simulink model "DDC_MPTC"  (R2023b)
settings: Solver=FixedStepDiscrete  StartTime=0.0  StopTime=0.5  RelTol=1e-3
libraries: spsGroundLib x1, spsPermanentMagnetSynchronousMachineLib x1, simulink x1, spsUniversalBridgeLib x1, spsDCVoltageSourceLib x1, slpidlib x1, spspowerguiLib x1
settings Model: Creator=蓝轩  LastModifiedBy=rainy
settings SolverCC: AlgebraicLoopSolver=TrustRegion
settings DataIOCC: ReturnWorkspaceOutputs=off
settings DebuggingCC: UnconnectedInputMsg=warning  UnconnectedOutputMsg=warning  UnconnectedLineMsg=warning  ArithmeticOperatorsInVariantConditions=warning
settings ModelReferenceCC: EnableRefExpFcnMdlSchedulingChecks=on
settings SFSimCC: CustomCodeUndefinedFunction=UseInterfaceOnly

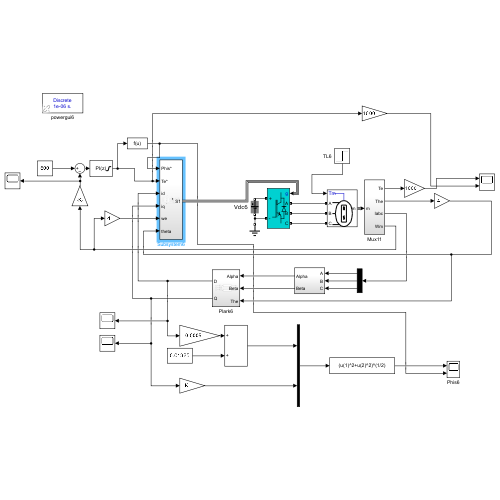
[thumbnail: Simulink's stored preview of the top-level diagram]
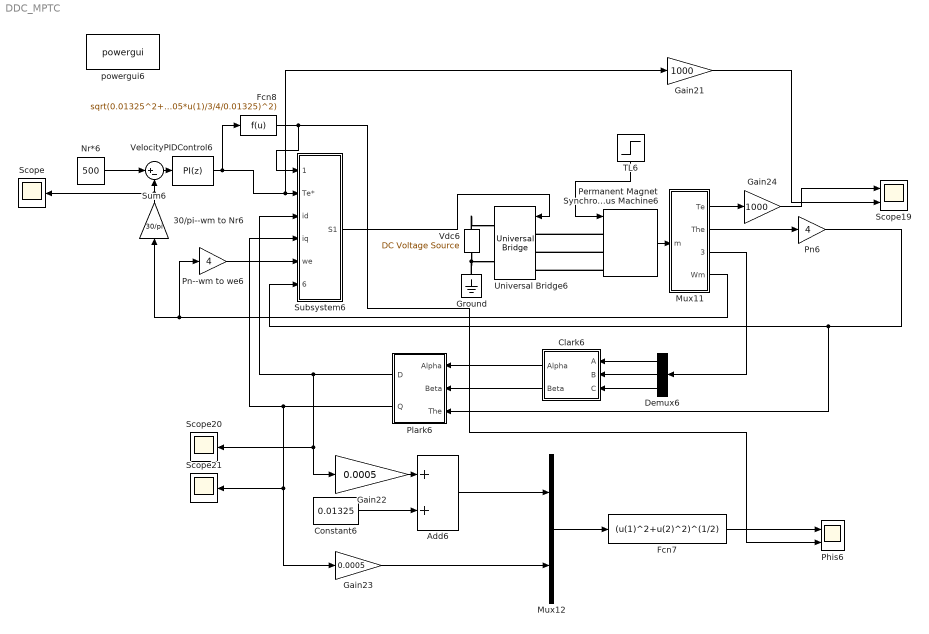
== system DDC_MPTC ==
  30/pi--wm to Nr6 : Gain  Gain=30/pi
  Add6 : Sum
  Clark6 : Subsystem
  Constant6 : Constant  Value=0.01325
  Demux6 : Demux  Outputs=3
  Fcn7 : Fcn  Expr=(u(1)^2+u(2)^2)^(1/2)
  Fcn8 : Fcn  Expr=sqrt(0.01325^2+(2*0.0005*u(1)/3/4/0.01325)^2)
  Gain21 : Gain  Gain=1000
  Gain22 : Gain  Gain=0.0005
  Gain23 : Gain  Gain=0.0005
  Gain24 : Gain  Gain=1000
  Ground : spsGroundLib/Ground  LConnTagsString=a
  Mux11 : Subsystem
  Mux12 : Mux  Inputs=2
  Nr*6 : Constant  Value=500
  Permanent Magnet Synchronous Machine6 : spsPermanentMagnetSynchronousMachineLib/Permanent Magnet Synchronous Machine  NbPhases=3  FluxDistribution=Sinusoidal  RotorType=Round  MechanicalLoad=Torque Tm  PresetModel=No  ShowDetailedParameters=on  MeasurementBus=off  Resistance=0.25  Inductance=8.5e-3  dqInductances=[8.5e-3,8.5e-3]  La=0.0005  MachineConstant=Flux linkage established by magnets (V.s)  Flux=0.01325  VoltageCst=9.6131  TorqueCst=0.0795  Flat=120  Mechanical=[0.00003 0 4 0]  PolePairs=4  InitialConditions=[0,0, 0,0]  InitialConditions5ph=[0 0 0 0 0 0]  RefAngle=Aligned with phase A axis (original Park)  IterativeDiscreteModel=Trapezoidal non iterative  TsBlock=-1  TsPowergui=0
  Phis6 : Scope  NumInputPorts=2
  Plark6 : Subsystem
  Pn--wm to we6 : Gain  Gain=4
  Pn6 : Gain  Gain=4
  Scope : Scope
  Scope19 : Scope  NumInputPorts=2
  Scope20 : Scope
  Scope21 : Scope
  Subsystem6 : Subsystem
  Sum6 : Sum  Inputs=|+-
  TL6 : Step  Time=0.25  Before=0.0  After=0.5
  Universal Bridge6 : spsUniversalBridgeLib/Universal Bridge  Arms=3  SnubberResistance=1e5  SnubberCapacitance=inf  Device=IGBT / Diodes  Ron=1e-3  Lon=0  ForwardVoltages="[  0  0  ]"  ForwardVoltage=0  GTOparameters=[ 10e-6 , 20e-6 ]  IGBTparameters=[ 1e-6 , 2e-6 ]  Measurements=None  Measurements_2=None  converterType=Rectifier
  Vdc6 : spsDCVoltageSourceLib/DC Voltage Source  Amplitude=24  Measurements=None
  VelocityPIDControl6 : slpidlib/PID Controller  Controller=PI  Form=Parallel  TimeDomain=Discrete-time  UseExternalTs=off  SampleTime=-1  IntegratorMethod=Forward Euler  FilterMethod=Forward Euler  ControllerParametersSource=internal  P=0.01  I=0.3  UseKiTs=off  D=0  N=100  UseFilter=on  TunerSelectOption=Transfer Function Based (PID Tuner App)  InitialConditionSource=internal  InitialConditionForIntegrator=0  InitialConditionForFilter=0  DifferentiatorICPrevScaledInput=0  ExternalReset=none  TrackingMode=off  Kt=1  LimitOutput=on  SatLimitsSource=internal  UpperSaturationLimit=1.27  LowerSaturationLimit=-1.27  LinearizeAsGain=on  AntiWindupMode=back-calculation  Kb=0.001  LimitIntegrator=off  UpperIntegratorSaturationLimit=inf  LowerIntegratorSaturationLimit=-inf  POutMin=[]  POutMax=[]  IOutMin=[]  IOutMax=[]  DOutMin=[]  DOutMax=[]  NOutMin=[]  NOutMax=[]  SumOutMin=[]  SumOutMax=[]  SaturationOutMin=[]  SaturationOutMax=[]  PParamMin=[]  PParamMax=[]  IParamMin=[]  IParamMax=[]  DParamMin=[]  DParamMax=[]  NParamMin=[]  NParamMax=[]  KbParamMin=[]  KbParamMax=[]  KtParamMin=[]  KtParamMax=[]  KbOutMin=[]  KbOutMax=[]  KtOutMin=[]  KtOutMax=[]  IntegratorOutMin=[]  IntegratorOutMax=[]  FilterOutMin=[]  FilterOutMax=[]  SumI1OutMin=[]  SumI1OutMax=[]  SumI2OutMin=[]  SumI2OutMax=[]  SumI3OutMin=[]  SumI3OutMax=[]  SumI4OutMin=[]  SumI4OutMax=[]  SumDOutMin=[]  SumDOutMax=[]  DifferentiatorOutMin=[]  DifferentiatorOutMax=[]  FilterDiffOutCoefMin=[]  FilterDiffOutCoefMax=[]  ReciprocalOutMin=[]  ReciprocalOutMax=[]  SumDenOutMin=[]  SumDenOutMax=[]  SumNumOutMin=[]  SumNumOutMax=[]  DivideOutMin=[]  DivideOutMax=[]  UdiffTsProdOutMin=[]  UdiffTsProdOutMax=[]  NTsProdOutMin=[]  NTsProdOutMax=[]  UintegralTsProdOutMin=[]  UintegralTsProdOutMax=[]  UngainTsProdOutMin=[]  UngainTsProdOutMax=[]  ClampingZeroOutDataTypeStr=Inherit: Inherit via back propagation  ClampingZeroOutMin=[]  ClampingZeroOutMax=[]  FilterDenConstantOutDataTypeStr=Inherit: Inherit via back propagation  FilterDenConstantOutMin=[]  FilterDenConstantOutMax=[]  PCopyOutDataTypeStr=Inherit: Inherit via back propagation  PCopyOutMin=[]  PCopyOutMax=[]  NCopyOutDataTypeStr=Inherit: Inherit via back propagation  NCopyOutMin=[]  NCopyOutMax=[]  IntegratorContinuousStateAttributes=''  IntegratorStateMustResolveToSignalObject=off  IntegratorRTWStateStorageClass=Auto  FilterContinuousStateAttributes=''  FilterStateMustResolveToSignalObject=off  FilterRTWStateStorageClass=Auto  ParallelPVariant=InternalParameters  IdealPVariant=Disabled  IVariant=InternalParameters  DVariant=Disabled  IntegratorVariant=Discrete  SatVariant=Enabled  AWVariant=BackCalculation  PCopyVariant=Disabled  TRVariant=Disabled  FdbkBlocksVariant=Forward  IdealPFdbkVariant=Disabled  SatFdbkVariant=Disabled  DerivativeFilterVariant=Disabled  NVariant=Disabled  NCopyVariant=Disabled_SignalSpec  FilterICVariant=Disabled  IntegratorICVariant=InternalICs  ExternalResetVariant=Disabled  TRSumVariant=Passthrough  SumFdbkVariant=Disabled  SumVariant=Sum_PI  TsampFilterVariant=InternalTs  TsampNgainVariant=Passthrough  TsampIntegralVariant=Disabled_SignalSpec  ExternalSaturationOutDataTypeStr=Inherit: Same as second input
  powergui6 : spspowerguiLib/powergui  Priority=1  SimulationMode=Discrete  SampleTime=0.000001  frequency=60  Iterations=50  frequencyindice=0  Pbase=100e6  ErrMax=1e-4  UnitsV=kV  UnitsW=MW  buscounter=0  FunctionMessages=off  echomessages=off  EnableUseOfTLC=off  CurrentSourceSwitches=off  DisableSnubberDevices=off  DisableRonSwitches=off  DisableVfSwitches=off  DisplayEquations=off  AutomaticDiscreteSolvers=off  SolverType=Tustin/Backward Euler (TBE)  Interpol=off  ExternalGateDelay=off  methode=off  Ts=100  x0status=blocks  SPID=off  SwTol=0  HookPort=off  NonlinearTolerance=1e-4  nMaxIteration=100  ContinueOnMaxIteration=off  RestoreLinks=warning  ResistiveCurrentMeasurement=off  Frange=[0:2:500]  Ylog=off  Xlog=on  ShowGrid=off  save=off  variable=ZData  structure=0  ZoomFFT=off  StartTime=0.0  cycles=1  DisplayStyle=1  fundamental=60  FreqAxis=off  MaxFrequency=1000  frequencyindicesteady=1  RmsSteady=1  display=off
  wires:
  Gain22/1 -> Add6/1
  Add6/1 -> Mux12/1
  Sum6/1 -> VelocityPIDControl6/1
  Nr*6/1 -> Sum6/1
  VelocityPIDControl6/1 -> Gain21/1, Subsystem6/2(Te*), Fcn8/1
  Mux12/1 -> Fcn7/1
  Mux11/2(The) -> Pn6/1
  TL6/1 -> Permanent Magnet Synchronous Machine6/1
  Clark6/1(Alpha) -> Plark6/1(Alpha)
  Fcn7/1 -> Phis6/1
  30/pi--wm to Nr6/1 -> Scope/1, Sum6/2
  Gain24/1 -> Scope19/1
  Mux11/1(Te) -> Gain24/1
  Clark6/2(Beta) -> Plark6/2(Beta)
  Constant6/1 -> Add6/2
  Pn--wm to we6/1 -> Subsystem6/5(we)
  Subsystem6/1(S1) -> Universal Bridge6/1
  Gain21/1 -> Scope19/2
  Gain23/1 -> Mux12/2
  Plark6/1(D) -> Scope20/1, Gain22/1, Subsystem6/3(id)
  Plark6/2(Q) -> Scope21/1, Gain23/1, Subsystem6/4(iq)
  Demux6/3 -> Clark6/3(C)
  Demux6/2 -> Clark6/2(B)
  Permanent Magnet Synchronous Machine6/1 -> Mux11/1(m)
  Pn6/1 -> Plark6/3(The), Subsystem6/6("theta ")
  Mux11/3(Iabc) -> Demux6/1
  Fcn8/1 -> Subsystem6/1(Phis*), Phis6/2
  Mux11/4(Wm) -> Pn--wm to we6/1, 30/pi--wm to Nr6/1
  Demux6/1 -> Clark6/1(A)
  connections:
  Vdc6/LConn1 -- Ground/LConn1 -- Universal Bridge6/RConn2
  Permanent Magnet Synchronous Machine6/LConn3 -- Universal Bridge6/LConn3
  Vdc6/RConn1 -- Universal Bridge6/RConn1
  Permanent Magnet Synchronous Machine6/LConn1 -- Universal Bridge6/LConn1
  Permanent Magnet Synchronous Machine6/LConn2 -- Universal Bridge6/LConn2

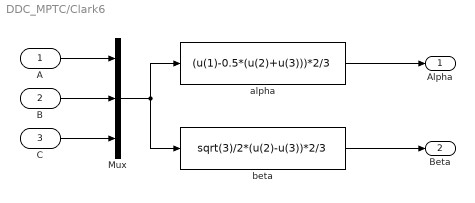
== system DDC_MPTC/Clark6 ==
  A : Inport
  B : Inport  Port=2
  C : Inport  Port=3
  Mux : Mux  Inputs=3
  alpha : Fcn  Expr=(u(1)-0.5*(u(2)+u(3)))*2/3
  beta : Fcn  Expr=sqrt(3)/2*(u(2)-u(3))*2/3
  Alpha : Outport  VectorParamsAs1DForOutWhenUnconnected=off
  Beta : Outport  Port=2  VectorParamsAs1DForOutWhenUnconnected=off
  wires:
  alpha/1 -> Alpha/1
  B/1 -> Mux/2
  C/1 -> Mux/3
  A/1 -> Mux/1
  Mux/1 -> beta/1, alpha/1
  beta/1 -> Beta/1

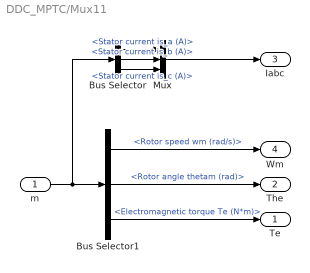
== system DDC_MPTC/Mux11 ==
  m : Inport
  Bus Selector : BusSelector  OutputSignals=Stator current is_a (A),Stator current is_b (A),Stator current is_c (A)
  Bus Selector1 : BusSelector  OutputSignals=Rotor speed wm (rad/s),Rotor angle thetam (rad),Electromagnetic torque Te (N*m)
  Mux : Mux  Inputs=3
  Te : Outport  VectorParamsAs1DForOutWhenUnconnected=off
  The : Outport  Port=2  VectorParamsAs1DForOutWhenUnconnected=off
  Iabc : Outport  Port=3  VectorParamsAs1DForOutWhenUnconnected=off
  Wm : Outport  Port=4  VectorParamsAs1DForOutWhenUnconnected=off
  wires:
  Bus Selector1/1 -> Wm/1  "<Rotor speed wm (rad/s)>"
  Bus Selector1/2 -> The/1  "<Rotor angle thetam (rad)>"
  Bus Selector1/3 -> Te/1  "<Electromagnetic torque Te (N*m)>"
  m/1 -> Bus Selector/1, Bus Selector1/1
  Bus Selector/2 -> Mux/2  "<Stator current is_b (A)>"
  Bus Selector/3 -> Mux/3  "<Stator current is_c (A)>"
  Bus Selector/1 -> Mux/1  "<Stator current is_a (A)>"
  Mux/1 -> Iabc/1

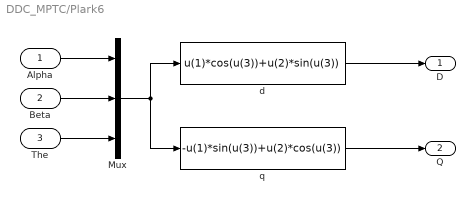
== system DDC_MPTC/Plark6 ==
  Alpha : Inport
  Beta : Inport  Port=2
  The : Inport  Port=3
  Mux : Mux  Inputs=3
  d : Fcn  Expr=u(1)*cos(u(3))+u(2)*sin(u(3))
  q : Fcn  Expr=-u(1)*sin(u(3))+u(2)*cos(u(3))
  D : Outport  VectorParamsAs1DForOutWhenUnconnected=off
  Q : Outport  Port=2  VectorParamsAs1DForOutWhenUnconnected=off
  wires:
  d/1 -> D/1
  Beta/1 -> Mux/2
  Alpha/1 -> Mux/1
  Mux/1 -> q/1, d/1
  q/1 -> Q/1
  The/1 -> Mux/3

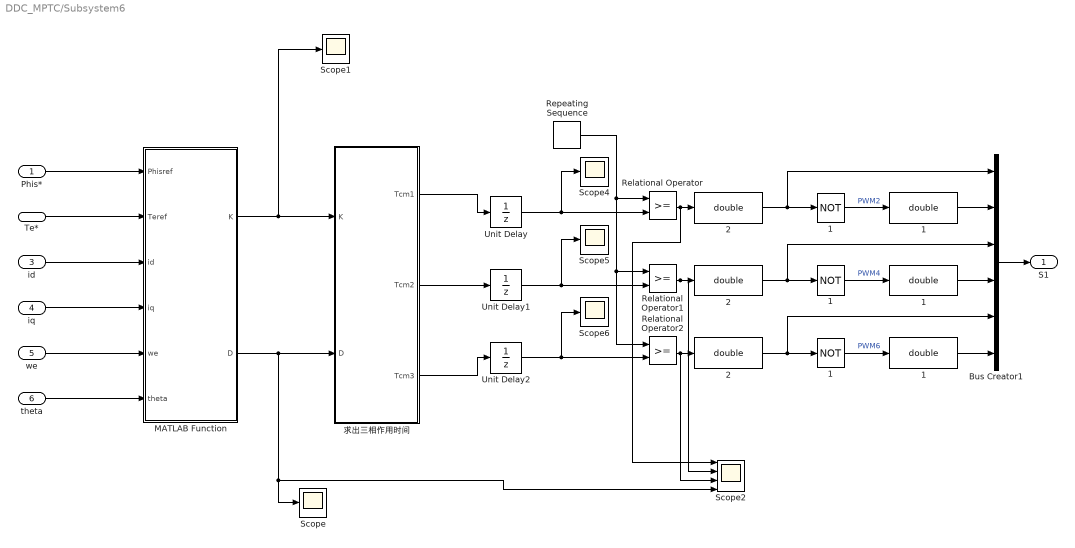
== system DDC_MPTC/Subsystem6 ==
  Phis* : Inport
  Te* : Inport  Port=2
  id : Inport  Port=3
  iq : Inport  Port=4
  we : Inport  Port=5
  "theta " : Inport  Port=6
  "         1" : DataTypeConversion  OutDataTypeStr=double  SaturateOnIntegerOverflow=off  RndMeth=Floor
  "         2" : DataTypeConversion  OutDataTypeStr=double  SaturateOnIntegerOverflow=off  RndMeth=Floor
  "       1" : Logic  Operator=NOT  AllPortsSameDT=off  OutDataTypeStr=boolean
  "     1" : DataTypeConversion  OutDataTypeStr=double  SaturateOnIntegerOverflow=off  RndMeth=Floor
  "     2" : DataTypeConversion  OutDataTypeStr=double  SaturateOnIntegerOverflow=off  RndMeth=Floor
  "   1" : Logic  Operator=NOT  AllPortsSameDT=off  OutDataTypeStr=boolean
  "  1" : DataTypeConversion  OutDataTypeStr=double  SaturateOnIntegerOverflow=off  RndMeth=Floor
  "  2" : DataTypeConversion  OutDataTypeStr=double  SaturateOnIntegerOverflow=off  RndMeth=Floor
  " 1" : Logic  Operator=NOT  AllPortsSameDT=off  OutDataTypeStr=boolean
  Bus Creator1 : BusCreator  Inputs=6
  MATLAB Function : MATLAB Function  TreatAsAtomicUnit=on
  Relational Operator : RelationalOperator  OutDataTypeStr=boolean  RndMeth=Simplest  InputSameDT=off
  Relational Operator1 : RelationalOperator  OutDataTypeStr=boolean  RndMeth=Simplest  InputSameDT=off
  Relational Operator2 : RelationalOperator  OutDataTypeStr=boolean  RndMeth=Simplest  InputSameDT=off
  Repeating Sequence : simulink/Sources/Repeating Sequence  rep_seq_t=[0 0.000025 0.00005]  rep_seq_y=[0 0.000025 0]
  Scope{,1,4..6} (5 alike) : Scope
  Scope2 : Scope  NumInputPorts=4
  Unit Delay : UnitDelay  SampleTime=0.00005  HasFrameUpgradeWarning=on
  Unit Delay1 : UnitDelay  SampleTime=0.00005  HasFrameUpgradeWarning=on
  Unit Delay2 : UnitDelay  SampleTime=0.00005  HasFrameUpgradeWarning=on
  求出三相作用时间 : MATLAB Function  TreatAsAtomicUnit=on
  S1 : Outport  VectorParamsAs1DForOutWhenUnconnected=off
  wires:
  Phis*/1 -> MATLAB Function/1(Phisref)
  Te*/1 -> MATLAB Function/2(Teref)
  id/1 -> MATLAB Function/3(id)
  iq/1 -> MATLAB Function/4(iq)
  we/1 -> MATLAB Function/5(we)
  "theta "/1 -> MATLAB Function/6(theta)
  MATLAB Function/1(K) -> Scope1/1, 求出三相作用时间/1(K)
  MATLAB Function/2(D) -> Scope2/4, Scope/1, 求出三相作用时间/2(D)
  求出三相作用时间/3(Tcm3) -> Unit Delay2/1
  "   1"/1 -> "     1"/1  "PWM4"
  "     2"/1 -> Bus Creator1/3, "   1"/1
  "     1"/1 -> Bus Creator1/4
  求出三相作用时间/1(Tcm1) -> Unit Delay/1
  " 1"/1 -> "  1"/1  "PWM2"
  Repeating Sequence/1 -> Relational Operator2/1, Relational Operator1/1, Relational Operator/1
  Relational Operator/1 -> Scope2/1, "  2"/1
  Relational Operator1/1 -> Scope2/2, "     2"/1
  求出三相作用时间/2(Tcm2) -> Unit Delay1/1
  "  1"/1 -> Bus Creator1/2
  "         2"/1 -> Bus Creator1/5, "       1"/1
  Relational Operator2/1 -> Scope2/3, "         2"/1
  "       1"/1 -> "         1"/1  "PWM6"
  "  2"/1 -> Bus Creator1/1, " 1"/1
  Bus Creator1/1 -> S1/1
  "         1"/1 -> Bus Creator1/6
  Unit Delay/1 -> Relational Operator/2, Scope4/1
  Unit Delay1/1 -> Scope5/1, Relational Operator1/2
  Unit Delay2/1 -> Relational Operator2/2, Scope6/1

== matlab function DDC_MPTC/Subsystem6/MATLAB Function ==
  settings: updateMethod=DISCRETE  sampleTime=0.00005
  data: Phisref input; Teref input; id input; iq input; we input; theta input; K output; D output
function [K,D]  = fcn(Phisref,Teref,id,iq,we,theta)

Ts=0.00005;R=0.25;Ld=0.0005;Lq=0.0005;Phif=0.01325;p=4;Vdc=24;gmin=20000000000000;m=250;K=1;D=1;

sw=[0 0 0;1 0 0;1 1 0;0 1 0;0 1 1;0 0 1;1 0 1;1 1 1];
trans=2/3*[cos(theta) cos(theta-2*pi/3) cos(theta+2*pi/3);-sin(theta) -sin(theta-2*pi/3) -sin(theta+2*pi/3)];


persistent M ud22 uq22 
if isempty(M)
    M=1; 
    ud22=0;  
    uq22=0; 
end

iq1=iq
id1=id
Te=3/2*p*iq1*Phif;
for i=1:8
      sa=sw(i,1);sb=sw(i,2);sc=sw(i,3);
      Va=(Vdc*(2*sa-sb-sc))/3;
      Vb=(Vdc*(2*sb-sa-sc))/3;   
      Vc=(Vdc*(2*sc-sb-sa))/3;
      Vabc=[Va;Vb;Vc];
      Vdq=trans*Vabc;
      Vd=Vdq(1,1);
      Vq=Vdq(2,1);
      idid=1/Ld*(Vd-R*id1+we*Lq*iq1)*Ts;
      iqid=1/Lq*(Vq-R*iq1-we*(Phif+Ld*id1))*Ts;
      idnext=id1+idid;
      iqnext=iq1+iqid;
      Tenext=3/2*p*iqnext*Phif;
      Phidnext=Ld*idnext+Phif;
      Phiqnext=Lq*iqnext;
      Phisnext=(Phidnext*Phidnext+Phiqnext*Phiqnext)^(1/2);
      
      ST0=1/Lq*(-R*iq1-we*(Phif+Ld*id1))*(3/2*p*Phif);
      STi=1/Lq*(Vq-R*iq1-we*(Phif+Ld*id1))*(3/2*p*Phif);
      Di=(Teref-Te-ST0*Ts)/(STi-ST0)/Ts;
      
      if(Di<=0||Di>=1)
          D_flag=100000;
          Di=1;
      else
          D_flag=0;
      end
      
      g=abs(Teref-Tenext)+m*abs(Phisref-Phisnext)+D_flag;
     
       if(g<gmin)
        K=i;
        D=Di;
        gmin=g;
      end
end

sa=sw(K,1);sb=sw(K,2);sc=sw(K,3);
Vamin=(Vdc*(2*sa-sb-sc))/3;
Vbmin=(Vdc*(2*sb-sa-sc))/3;   
Vcmin=(Vdc*(2*sc-sb-sa))/3;
Vabcmin=[Vamin;Vbmin;Vcmin];
Vdqmin=trans*Vabcmin;
ud22=Vdqmin(1,1)*D;
uq22=Vdqmin(2,1)*D;

== matlab function DDC_MPTC/Subsystem6/求出三相作用时间 ==
  settings: updateMethod=DISCRETE  sampleTime=0.00005
  data: K input; Tcm1 output; D input; Tcm2 output; Tcm3 output
function [Tcm1,Tcm2,Tcm3] = fcn(K,D)

Ts=0.00005;

T1=D*Ts/2;
T2=T1;
Ta=(Ts-T1-T2)/4;
Tb=Ta+T1/2;
Tc=Tb+T2/2;
Tcm1=1;
Tcm2=1;
Tcm3=1;

if(K==1)
    Tcm1=Tc;Tcm2=Tc;Tcm3=Tc;
end
if(K==2) 
    Tcm1=Ta;Tcm2=Tc;Tcm3=Tc;
end
if(K==3) 
    Tcm1=Ta;Tcm2=Ta;Tcm3=Tc;
end
if(K==4) 
    Tcm1=Tc;Tcm2=Ta;Tcm3=Tc;
end
if(K==5) 
    Tcm1=Tc;Tcm2=Ta;Tcm3=Ta;
end
if(K==6) 
    Tcm1=Tc;Tcm2=Tc;Tcm3=Ta;
end
if(K==7) 
    Tcm1=Ta;Tcm2=Tc;Tcm3=Ta;
end
if(K==8)
    Tcm1=Ta;Tcm2=Ta;Tcm3=Ta;
end
